simulink model "ftm_hall_sensor_s32k14x"  (Simulink 9.0)
settings: Solver=FixedStepDiscrete  StartTime=0.0  StopTime=20.0  FixedStep=0.001  RelTol=1e-3  EnableMultiTasking=on
model workspace (MAT data in the model file):
  ClockFreq = Simulink.Parameter
  ClockFreq.Value = 80000000
  ClockFreq.Description = 'FTM Input Clock Frequency'
  ClockFreq.DataType = 'single'
  ClockFreq.Min = 0
  ClockFreq.Dimensions = [1 1]
  ClockPrescaler = Simulink.Parameter
  ClockPrescaler.Value = 128
  ClockPrescaler.Description = 'FTM Clock Prescaler set in the Simulink Block'
  ClockPrescaler.DataType = 'single'
  ClockPrescaler.Min = 1
  ClockPrescaler.Max = 128
  ClockPrescaler.Dimensions = [1 1]
  EdgeMode = Simulink.Parameter
  EdgeMode.Value = 1
  EdgeMode.Description = 'Edge Mode parameter:
    | - Rising = 2
    | - Falling = 2
    | - Rising or Falling = 1'
  EdgeMode.DataType = 'auto'
  EdgeMode.Min = 1
  EdgeMode.Max = 2
  EdgeMode.Dimensions = [1 1]
  NoHallsTrans = Simulink.Parameter
  NoHallsTrans.Value = 6
  NoHallsTrans.DataType = 'single'
  NoHallsTrans.Min = 1
  NoHallsTrans.Dimensions = [1 1]
  PP = Simulink.Parameter
  PP.Value = 2
  PP.Description = 'Motor number of Pole Pairs'
  PP.DataType = 'single'
  PP.Min = 0
  PP.Dimensions = [1 1]
InitFcn:
  | mbd_s32k_consistency_checks(bdroot(gcs));
undefined symbols (not defined in the file): LQFP
libraries: mbd_s32k1xx_ec_toolbox x8, dspstat3 x1, simulink x1
Description:
  | This model shows FlexTimer's Hall Sensor.
  | 
  | The Hall sensors signals of a running motor are emulated using the block
  | called Hall_Sensor_signals_generation by toggling the output of the pins
  | PTB14, PTB15, and PTB16 using the GPIO.
  | 
  | The FTM Hall sensor block has as input the pins PTA1, PTD10, and PTD11.
  | 
  | For the example to work, connect the emulated signals Hall sensors to input
  | pins of FTM Hall sensor block, for example connect PTB14 to PTA1, PTB15 to
  | PTD10, and PTB16 to PTD11.
  | 
  | This example has also a FreeMaster project associated, which is called
  | "ftm_hall_sensor_s32k14x.pmp". The project has a scope called "Speed
  | Computation" and a recorder called "Sensors".
  | 
  | For a given value of "Speed_Command" variable the pins PTB14, PTB15, and
  | PTB16 will be the same values as the signals of Hall sensors of a spinning
  | motor at the speed "Speed_Command". It's value can be modified from
  | FreeMaster.
  | 
  | Validation: In FreeMaster "Motor_Speed" should be equal to "Speed_Command".
settings Model: Creator=NXP MBDT Team  LastModifiedBy=nxf35172
settings DataIOCC: ExternalInput=off  InitialState=off  LimitDataPoints=on  SaveOutput=off  SignalLogging=off  SaveTime=off
settings OptimizationCC: DefaultParameterBehavior=Inlined  LifeSpan=1
settings DebuggingCC: SolverPrmCheckMsg=warning  InheritedTsInSrcMsg=none  SingleTaskRateTransMsg=error  UnconnectedInputMsg=error  UnconnectedOutputMsg=error  UnconnectedLineMsg=error  AllowSymbolicDim=off  UnknownTsInhSupMsg=error  StateNameClashWarn=warning
settings HardwareCC: ProdLargestAtomicInteger=Long  ProdLargestAtomicFloat=Double  ProdEndianess=LittleEndian  ProdHWDeviceType=ARM Compatible->ARM Cortex
settings SFSimCC: MATLABDynamicMemAlloc=off
settings RTWCC: SystemTargetFile=mbd_s32k.tlc  MakeCommand=mbd_s32k_make_rtw COPY_MDLREF_INCLUDES=0  TemplateMakefile=mbd_s32k.tmf  Description=Model Based Design Toolbox S32K14x Code Generation Target  GenerateReport=on  LaunchReport=on
settings CodeAppCC: IgnoreCustomStorageClasses=off
settings STFCustomTargetCC: CombineOutputUpdateFcns=on  ERTCustomFileBanners=on  SupportContinuousTime=off  SupportNonInlinedSFcns=off  RemoveResetFunc=on  MATLABClassNameForMDSCustomization=Simulink.SoftwareTarget.ERTCustomization  GRTInterface=off  SystemTargetFile=mbd_s32k14.tlc
settings ERTTargetCC: MultiwordLength=2048  ParMdlRefBuildCompliant=off  CompOptLevelCompliant=off  ConcurrentExecutionCompliant=off  ModelStepFunctionPrototypeControlCompliant=off  CPPClassGenCompliant=off  UseToolchainInfoCompliant=off  InlinedParameterPlacement=NonHierarchical  ERTCustomFileTemplate=example_file_process.tlc  ConvertIfToSwitch=off  SuppressUnreachableDefaultCases=off

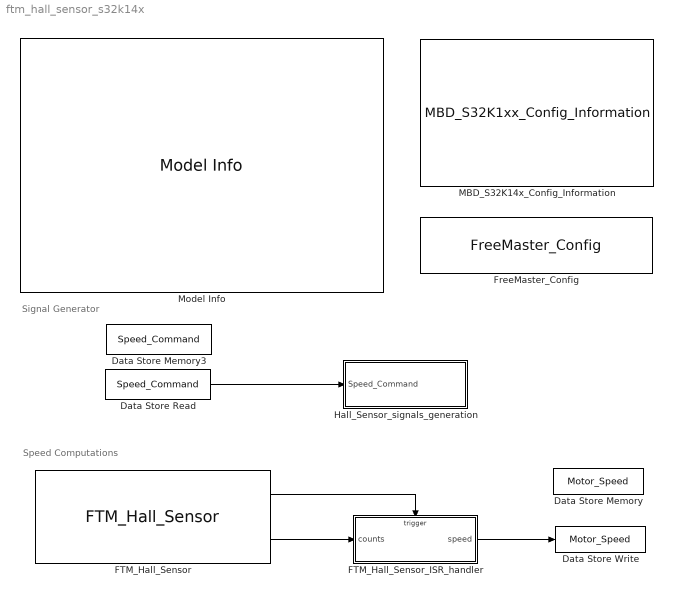
== system ftm_hall_sensor_s32k14x ==
  note: Speed Computations
  note: Signal Generator
  Data Store Memory : DataStoreMemory  DataStoreName=Motor_Speed  ReadBeforeWriteMsg=warning  WriteAfterWriteMsg=warning  WriteAfterReadMsg=warning  ShowAdditionalParam=off  OutDataTypeStr=single
  Data Store Memory3 : DataStoreMemory  DataStoreName=Speed_Command  ReadBeforeWriteMsg=warning  WriteAfterWriteMsg=warning  WriteAfterReadMsg=warning  InitialValue=1000  ShowAdditionalParam=off  OutDataTypeStr=single
  Data Store Read : DataStoreRead  DataStoreName=Speed_Command
  Data Store Write : DataStoreWrite  DataStoreName=Motor_Speed  DataStoreElements=Motor_Speed
  FTM_Hall_Sensor : mbd_s32k1xx_ec_toolbox/Motor Control Blocks/FTM Blocks/FTM_Hall_Sensor  Priority=1  e_mode=Rising or Falling  prescaler=128  max_period=0.10486  isrlevel=2  mcuTargetUpdate=on  filter_en=off  filter_value=0  pinFtm1Ch1=PTA1: [FTM1_CH1 | FTM Channel]  pinFtm2Ch0=PTD10: [FTM2_CH0 | FTM Channel]  pinFtm2Ch1=PTD11: [FTM2_CH1 | FTM Channel]
  FTM_Hall_Sensor_ISR_handler : Subsystem  TreatAsAtomicUnit=on
      settings: RTWSystemCode=Nonreusable function
  FreeMaster_Config : mbd_s32k1xx_ec_toolbox/Utility Blocks/FreeMaster_Config  interface=LPUART1  baudrate=115200  rxd=PTC6: [LPUART1_RX | Receive]  txd=PTC7: [LPUART1_TX | Transmit]  mode=Short Interrupt  isr_prio=10  show_adv_opts=on  use_scope=on  max_scope_vars=8  use_recorder=on  max_rec_vars=8  rec_buff_size=1024  rec_timebase=10 milliseconds  comm_buffer_size_auto=on  comm_buffer_size=255  comm_rqueue_size_default=on  comm_rqueue_size=32
  Hall_Sensor_signals_generation : Subsystem  TreatAsAtomicUnit=on
      settings: RTWSystemCode=Nonreusable function
  MBD_S32K14x_Config_Information : mbd_s32k1xx_ec_toolbox/MBD_S32K1xx_Config_Information  mbdt_ver=0  disp_str=|  config_params=[]  mcu_target_name=S32K146  mcu_target_package=64-LQFP  mcu_target_sram_size=128KB  mcu_system_clock_freq=80  mcu_xtal_freq=External 8  mcu_steptick_timer=LPIT Channel 0  mcu_steptick_prio=15  ds_import_enable=on  target_compiler=GCC  target_memory=FLASH  gcc_target_compile_opts=-mcpu=cortex-m4 -mthumb -mfloat-abi=hard -mfpu=fpv4-sp-d16 -O1 -g -gstrict-dwarf  gcc_target_assemble_opts=-mcpu=cortex-m4 -mthumb -mfloat-abi=hard -mfpu=fpv4-sp-d16 -g  gcc_target_link_opts=-mcpu=cortex-m4 -mthumb -mfloat-abi=hard -mfpu=fpv4-sp-d16  gcc_target_default_lcf=on  gcc_target_user_lcf=S32K146_128_flash.ld  ghs_target_compile_opts=-cpu=cortexm4f -thumb -DARM_MATH_CM4 -fpu=vfpv4_d16 -fsingle -Ogeneral -Wundef -Wimplicit-int -Wshadow -Wtrigraphs --no_commons --gnu_asm -gnu99 -gdwarf-2 -G  ghs_target_assemble_opts=-cpu=cortexm4f -fpu=vfpv4_d16  ghs_target_link_opts=-cpu=cortexm4f -thumb -fpu=vfpv4_d16  ghs_target_default_lcf=off  ghs_target_user_lcf=S32K146_128_flash.ld  iar_target_compile_opts=--cpu=Cortex-M4F --thumb --fpu=VFPv4_sp -Ol -e --debug --dlib_config normal  iar_target_assemble_opts=--cpu Cortex-M4F --thumb --fpu VFPv4_sp  iar_target_link_opts=--no_exceptions --vfe --inline  iar_target_default_lcf=off  iar_target_user_lcf=S32K146_128_flash.icf  pil_download_enable=off  rbl_download_enable=on  rbl_start_delay=5000000  rbl_download_interface=OpenSDA  rbl_restart_request=off  rbl_com_port=Custom  rbl_com_port_custom=COM1  pil_download_rate=57600  pil_opensda_drive=Custom  pil_opensda_drive_custom=E  pil_uart_instance=0  pil_uart_rx=PTA2: [LPUART0_RX | Receive]  pil_uart_tx=PTA3: [LPUART0_TX | Transmit]  FTM_PWM_PcrCheckEnDis=on  FTM_Input_Edge_Inputs_PcrCheckEnDis=on  FTM_Dual_Edge_Inputs_PcrCheckEnDis=on  FTM_Quadrature_Inputs_PcrCheckEnDis=on  FTM_Hall_Sensor_Inputs_PcrCheckEnDis=on  LPTMR_PcrCheckEnDis=on  PIT_PcrCheckEnDis=on  RTC_PcrCheckEnDis=on  FlexCAN_PcrCheckEnDis=on  LIN_PcrCheckEnDis=on  FlexIO_PcrCheckEnDis=on  LPI2C_PcrCheckEnDis=on  LPSPI_PcrCheckEnDis=on  LPUART_PcrCheckEnDis=on  CMP_PcrCheckEnDis=on  GPIO_OutputPcrCheckEnDis=on  GPIO_InputPcrCheckEnDis=on  SBC_PcrCheckEnDis=on  AMMCLIB_PcrCheckEnDis=on  FM_PcrCheckEnDis=on  Profile_PcrCheckEnDis=on  ConfigParams_PcrCheckEnDis=on  ModelRef_PcrCheckEnDis=on  PDB0_PcrCheckEnDis=on  CSEc_PcrCheckEnDis=on  eDMA_PcrCheckEnDis=on  ADC_PcrCheckEnDis=on  WDOG_PcrCheckEnDis=on
      | Target : S32K142-16KB_SRAM
      | Package : 100-pin
      | System clock : 80 MHz
      | XTAL clock : External 8 MHz
      | Compiler : GCC
      | Target Type : FLASH
      | Download Code after build : (OpenSDA: E)
      | Step Tick Interrupt Priority : 15
  Model Info : simulink/Model-Wide Utilities/Model Info  Frame=off  DisplayStringWithTags=|  HorizontalTextAlignment=Left  LeftAlignmentValue=0.02
      | Model Name: %<ModelName>
      | 
      | Description: %<Description>
  wires:
  FTM_Hall_Sensor/1 -> FTM_Hall_Sensor_ISR_handler/Trigger
  FTM_Hall_Sensor_ISR_handler/1(speed) -> Data Store Write/1
  FTM_Hall_Sensor/2 -> FTM_Hall_Sensor_ISR_handler/1(counts)
  Data Store Read/1 -> Hall_Sensor_signals_generation/1(Speed_Command)

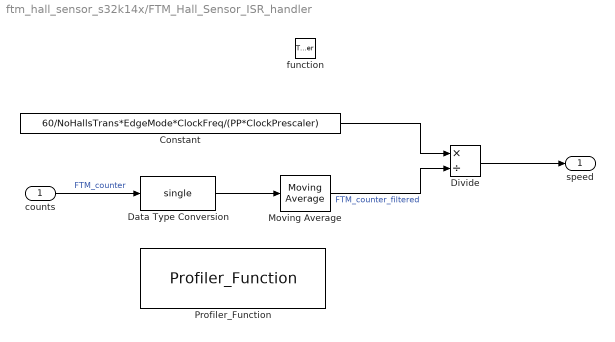
== system ftm_hall_sensor_s32k14x/FTM_Hall_Sensor_ISR_handler ==
  counts : Inport
  function : TriggerPort  TriggerType=function-call  VariantControl=Variant
  Constant : Constant  Value=60/NoHallsTrans*EdgeMode*ClockFreq/(PP*ClockPrescaler)  OutDataTypeStr=single
  Data Type Conversion : DataTypeConversion  OutDataTypeStr=single
  Divide : Product  Inputs=*/
  Moving Average : dspstat3/Moving Average  Method=Sliding window  SpecifyWindowLength=on  WindowLength=12  ForgettingFactor=0.9  SimulateUsing=Code generation
  Profiler_Function : mbd_s32k1xx_ec_toolbox/Utility Blocks/Profiler_Function  profile_indx=0
  speed : Outport
  wires:
  Divide/1 -> speed/1
  Constant/1 -> Divide/1
  Data Type Conversion/1 -> Moving Average/1
  Moving Average/1 -> Divide/2  "FTM_counter_filtered"
  counts/1 -> Data Type Conversion/1  "FTM_counter"

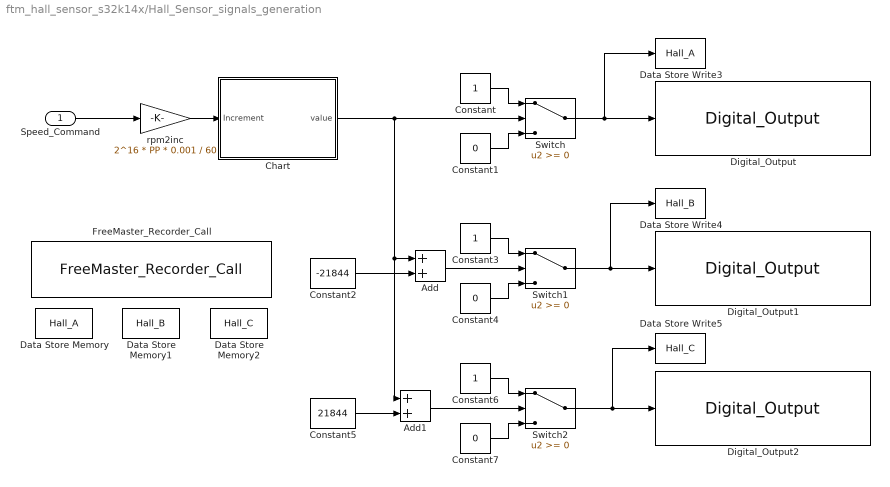
== system ftm_hall_sensor_s32k14x/Hall_Sensor_signals_generation ==
  Speed_Command : Inport
  Add : Sum
  Add1 : Sum
  Chart : Stateflow chart  TreatAsAtomicUnit=on
  Constant : Constant
  Constant1 : Constant  Value=0
  Constant2 : Constant  Value=-21844  OutDataTypeStr=int16
  Constant3 : Constant
  Constant4 : Constant  Value=0
  Constant5 : Constant  Value=21844  OutDataTypeStr=int16
  Constant6 : Constant
  Constant7 : Constant  Value=0
  Data Store Memory : DataStoreMemory  DataStoreName=Hall_A  ReadBeforeWriteMsg=warning  WriteAfterWriteMsg=warning  WriteAfterReadMsg=warning  ShowAdditionalParam=off  OutDataTypeStr=boolean
  Data Store Memory1 : DataStoreMemory  DataStoreName=Hall_B  ReadBeforeWriteMsg=warning  WriteAfterWriteMsg=warning  WriteAfterReadMsg=warning  ShowAdditionalParam=off  OutDataTypeStr=boolean
  Data Store Memory2 : DataStoreMemory  DataStoreName=Hall_C  ReadBeforeWriteMsg=warning  WriteAfterWriteMsg=warning  WriteAfterReadMsg=warning  ShowAdditionalParam=off  OutDataTypeStr=boolean
  Data Store Write3 : DataStoreWrite  DataStoreName=Hall_A
  Data Store Write4 : DataStoreWrite  DataStoreName=Hall_B
  Data Store Write5 : DataStoreWrite  DataStoreName=Hall_C
  Digital_Output : mbd_s32k1xx_ec_toolbox/GPIO Blocks/Digital_Output  gpio_pin=PTB14: [PTB14 | Port B I/O]  init_val=Low  drive_strength=Low
  Digital_Output1 : mbd_s32k1xx_ec_toolbox/GPIO Blocks/Digital_Output  gpio_pin=PTB15: [PTB15 | Port B I/O]  init_val=Low  drive_strength=Low
  Digital_Output2 : mbd_s32k1xx_ec_toolbox/GPIO Blocks/Digital_Output  gpio_pin=PTB16: [PTB16 | Port B I/O]  init_val=Low  drive_strength=Low
  FreeMaster_Recorder_Call : mbd_s32k1xx_ec_toolbox/Utility Blocks/FreeMaster_Recorder_Call
  Switch : Switch  OutDataTypeStr=Inherit: Inherit via back propagation
  Switch1 : Switch  OutDataTypeStr=Inherit: Inherit via back propagation
  Switch2 : Switch  OutDataTypeStr=Inherit: Inherit via back propagation
  rpm2inc : Gain  Gain=2^16 * PP * 0.001 / 60  OutDataTypeStr=Inherit: Inherit via back propagation
  wires:
  Chart/1(value) -> Add1/1, Add/1, Switch/2
  Speed_Command/1 -> rpm2inc/1
  Constant/1 -> Switch/1
  Constant1/1 -> Switch/3
  Constant7/1 -> Switch2/3
  Add1/1 -> Switch2/2
  Constant2/1 -> Add/2
  Add/1 -> Switch1/2
  Constant3/1 -> Switch1/1
  Constant5/1 -> Add1/2
  Constant6/1 -> Switch2/1
  Constant4/1 -> Switch1/3
  Switch1/1 -> Data Store Write4/1, Digital_Output1/1
  Switch2/1 -> Data Store Write5/1, Digital_Output2/1
  Switch/1 -> Data Store Write3/1, Digital_Output/1
  rpm2inc/1 -> Chart/1(Increment)

== stateflow chart Hall_Sensor_signals_generation/Chart ==
  settings: executeAtInitialization=1
  state A
    du:
    cntr=cntr+Increment;
    value=cntr;
    ex:
    cntr = -32767;
  (default) -> A : {cntr=0;}
  A -> A : [cntr >= 32767]
  data: cntr local int16 =0; value output int16; Increment input int16
